simulink model "P6SLink"  (R2026a)
settings: Solver=VariableStepAuto  StopTime=0.005  MaxStep=1e-6

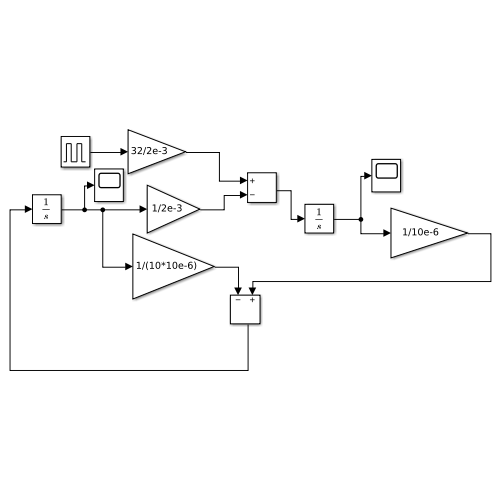
[thumbnail: Simulink's stored preview of the top-level diagram]
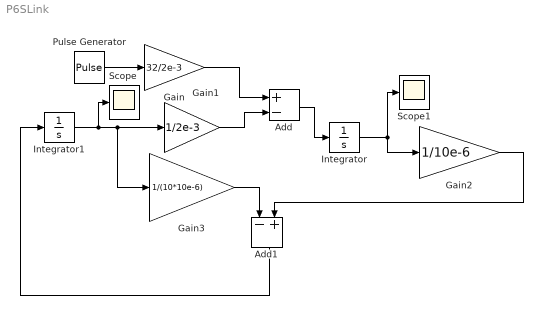
== system P6SLink ==
  Add : Sum  Inputs=+-
  Add1 : Sum  Inputs=-+
  Gain : Gain  Gain=32/2e-3
  Gain1 : Gain  Gain=1/2e-3
  Gain2 : Gain  Gain=1/10e-6
  Gain3 : Gain  Gain=1/(10*10e-6)
  Integrator : Integrator
  Integrator1 : Integrator
  Pulse Generator : DiscretePulseGenerator  PulseType=Time based  Period=1/100e3  PulseWidth=40
  Scope : Scope
      settings: ActiveDisplayYMinimum=-1.669429266955462  ActiveDisplayYMaximum=15.024863402599163
  Scope1 : Scope
      settings: ActiveDisplayYMinimum=-0.17312047082287454  ActiveDisplayYMaximum=1.5580842374058712
  wires:
  Pulse Generator/1 -> Gain/1
  Integrator1/1 -> Scope/1, Gain3/1, Gain1/1
  Gain/1 -> Add/1
  Gain1/1 -> Add/2
  Integrator/1 -> Gain2/1, Scope1/1
  Add/1 -> Integrator/1
  Add1/1 -> Integrator1/1
  Gain3/1 -> Add1/1
  Gain2/1 -> Add1/2
